simulink model "IRISC_control_model"  (R2015b)
settings: Solver=ode4  StartTime=0.0  StopTime=t_end  FixedStep=dt_sim  RelTol=1e-3
values from neighbouring files (symbols this model uses):
  dt_control = 1/50    (= 0.02)    [initialize_params.m]
  dt_gyr = 1/f_gyr    (= 0.02)    [initialize_params.m]
  dt_str = 5    [illustrate_kalman_filter.m]    (also in initialize_params.m)
  gyr_delay = 2*dt_gyr    (= 0.04)    [initialize_params.m]
  gyro_bias_0 = 10/180*pi/3600    (= 4.8481368111e-05)    [illustrate_kalman_filter.m]    (also in initialize_params.m)
  I_el = 5    [initialize_params.m]
  Kd = I_el*2*zeta*wn    (= 0.188495559215)    [initialize_params.m]
  Ki = I_el*(wn^2/T)    (= 1.11622596049e-05)    [initialize_params.m]
  Kp = I_el*wn^2    (= 0.0017765287922)    [initialize_params.m]
  Tmax = .1    (= 0.1)    [initialize_params.m]
libraries: simulink x2
settings Model: Creator=jeroenvandersteen  LastModifiedBy=jeroenvandersteen

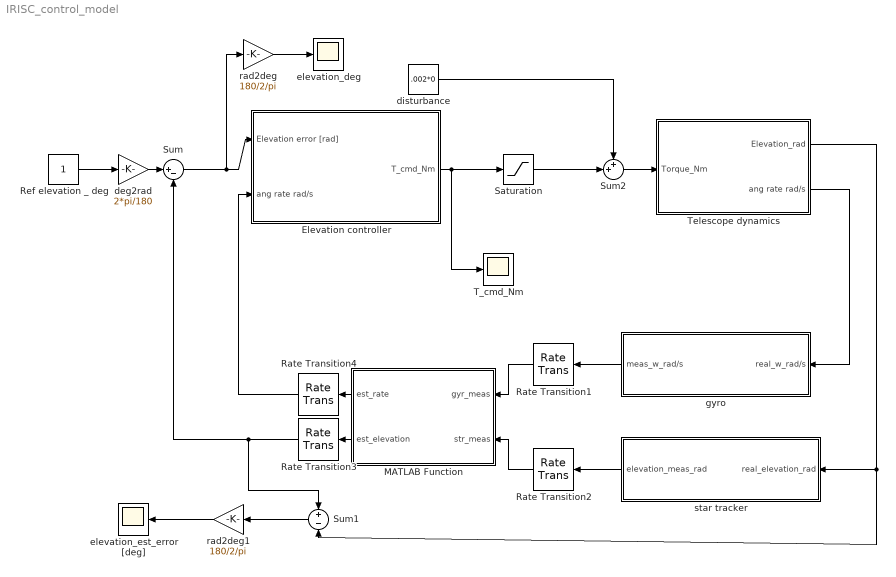
== system IRISC_control_model ==
  Elevation controller : Subsystem
  MATLAB Function : MATLAB Function  TreatAsAtomicUnit=on  SystemSampleTime=dt_control
  Rate Transition{1..4} (4 alike) : RateTransition
  Ref elevation _ deg : Constant
  Saturation : Saturate  UpperLimit=Tmax  LowerLimit=-Tmax
  Sum : Sum  Inputs=|+-
  Sum1 : Sum  Inputs=+-
  Sum2 : Sum  Inputs=++|
  T_cmd_Nm : Scope
  Telescope dynamics : Subsystem
  deg2rad : Gain  Gain=2*pi/180
  disturbance : Constant  Value=.002*0
  elevation_deg : Scope
  elevation_est_error [deg] : Scope
  gyro : Subsystem
  rad2deg : Gain  Gain=180/2/pi
  rad2deg1 : Gain  Gain=180/2/pi
  star tracker : Subsystem
  wires:
  Ref elevation _ deg/1 -> deg2rad/1
  deg2rad/1 -> Sum/1
  Sum/1 -> Elevation controller/1(Elevation error [rad]), rad2deg/1
  rad2deg/1 -> elevation_deg/1
  Sum2/1 -> Telescope dynamics/1(Torque_Nm)
  disturbance/1 -> Sum2/1
  Elevation controller/1(T_cmd_Nm) -> T_cmd_Nm/1, Saturation/1
  Saturation/1 -> Sum2/2
  Telescope dynamics/1(Elevation_rad) -> star tracker/1(real_elevation_rad), Sum1/2
  Telescope dynamics/2(ang rate rad/s) -> gyro/1(real_w_rad/s)
  gyro/1(meas_w_rad/s) -> Rate Transition1/1
  star tracker/1(elevation_meas_rad) -> Rate Transition2/1
  MATLAB Function/1(est_rate) -> Rate Transition4/1
  MATLAB Function/2(est_elevation) -> Rate Transition3/1
  Sum1/1 -> rad2deg1/1
  rad2deg1/1 -> elevation_est_error [deg]/1
  Rate Transition1/1 -> MATLAB Function/1(gyr_meas)
  Rate Transition2/1 -> MATLAB Function/2(str_meas)
  Rate Transition3/1 -> Sum1/1, Sum/2
  Rate Transition4/1 -> Elevation controller/2(ang rate rad/s)

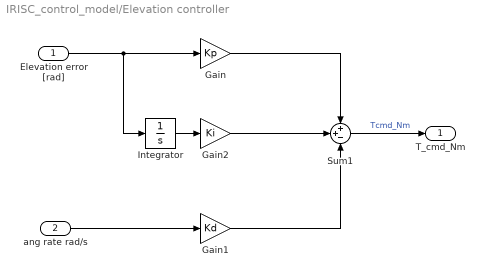
== system IRISC_control_model/Elevation controller ==
  Elevation error [rad] : Inport
  ang rate rad/s : Inport  Port=2
  Gain : Gain  Gain=Kp
  Gain1 : Gain  Gain=Kd
  Gain2 : Gain  Gain=Ki
  Integrator : Integrator
  Sum1 : Sum  Inputs=++-
  T_cmd_Nm : Outport
  wires:
  Sum1/1 -> T_cmd_Nm/1  "Tcmd_Nm"
  ang rate rad/s/1 -> Gain1/1
  Elevation error [rad]/1 -> Integrator/1, Gain/1
  Integrator/1 -> Gain2/1
  Gain2/1 -> Sum1/2
  Gain/1 -> Sum1/1
  Gain1/1 -> Sum1/3

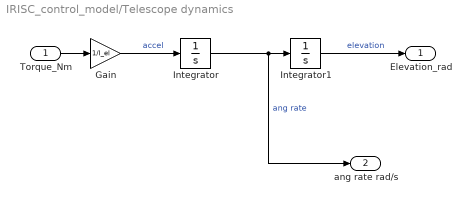
== system IRISC_control_model/Telescope dynamics ==
  Torque_Nm : Inport
  Gain : Gain  Gain=1/I_el
  Integrator : Integrator
  Integrator1 : Integrator
  Elevation_rad : Outport
  ang rate rad/s : Outport  Port=2
  wires:
  Torque_Nm/1 -> Gain/1
  Integrator1/1 -> Elevation_rad/1  "elevation"
  Gain/1 -> Integrator/1  "accel"
  Integrator/1 -> ang rate rad/s/1, Integrator1/1  "ang rate"

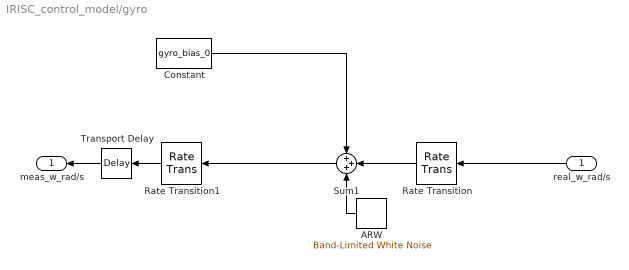
== system IRISC_control_model/gyro ==
  real_w_rad/s : Inport
  ARW : simulink/Sources/Band-Limited White Noise  Cov=PSD_gyr  Ts=dt_gyr  seed=[23341]
  Constant : Constant  Value=gyro_bias_0
  Rate Transition : RateTransition
  Rate Transition1 : RateTransition
  Sum1 : Sum  Inputs=+++
  Transport Delay : TransportDelay  DelayTime=gyr_delay
  meas_w_rad/s : Outport
  wires:
  Rate Transition1/1 -> Transport Delay/1
  real_w_rad/s/1 -> Rate Transition/1
  Rate Transition/1 -> Sum1/2
  ARW/1 -> Sum1/3
  Constant/1 -> Sum1/1
  Transport Delay/1 -> meas_w_rad/s/1
  Sum1/1 -> Rate Transition1/1

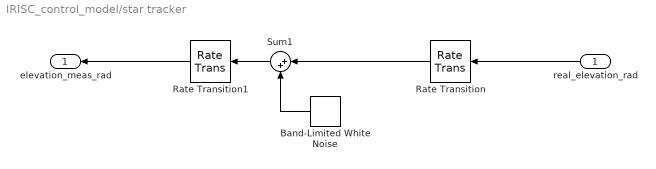
== system IRISC_control_model/star tracker ==
  real_elevation_rad : Inport
  Band-Limited White Noise : simulink/Sources/Band-Limited White Noise  Cov=PSD_str  Ts=dt_str  seed=[23341]
  Rate Transition : RateTransition
  Rate Transition1 : RateTransition
  Sum1 : Sum  Inputs=|++
  elevation_meas_rad : Outport
  wires:
  real_elevation_rad/1 -> Rate Transition/1
  Sum1/1 -> Rate Transition1/1
  Band-Limited White Noise/1 -> Sum1/2
  Rate Transition/1 -> Sum1/1
  Rate Transition1/1 -> elevation_meas_rad/1

== matlab function IRISC_control_model/MATLAB Function ==
  data: est_rate output; gyr_meas input; str_meas input; est_elevation output
function [est_rate,est_elevation] = estimator(gyr_meas,str_meas)
%#codegen

dt_control = 1/50;
tol = 1e-12;

persistent prev_str_meas;
persistent prev_elev_est;

if isempty(prev_str_meas);
    prev_str_meas = str_meas;
end
if isempty(prev_elev_est);
    prev_elev_est = str_meas;
end

if abs(str_meas - prev_str_meas) < tol
    est_elevation = prev_elev_est + dt_control*gyr_meas;
else
    est_elevation = str_meas;
end
prev_elev_est = est_elevation;
prev_str_meas = str_meas;

est_rate = gyr_meas;
est_elevation = str_meas;
